simulink model "Pendule_Observateur_Controleur_Discret"  (Simulink 8.4)
settings: Solver=ode3  StartTime=0.0  StopTime=10.0  RelTol=1e-3
values from neighbouring files (symbols this model uses):
  A = zeros (4,4)    [Modele_Pendule.m]
  Aod = Ad-Kod*Cd    [Design_Matlab_File_Pendule_IMC_.m]
  B = zeros (4,1)    [Modele_Pendule.m]
  Bod = [Bd Kod]    [Design_Matlab_File_Pendule_IMC_.m]
  C = [1 0 0 0 ... (first row only)    [Modele_Pendule.m]
  Cod = eye(4,4)    [Design_Matlab_File_Pendule_IMC_.m]
  D = [ 0 0 ]'    [Modele_Pendule.m]
  Dod = zeros(4,3)    [Design_Matlab_File_Pendule_IMC_.m]
  Kcd = place(Ad,Bd,Pcd)    [Design_Matlab_File_Pendule_IMC_.m]
  T_ech = 0.005    [Design_Matlab_File_Pendule_IMC_.m]
  X0 = [0.3 0 0 0]'    [Design_Matlab_File_Pendule_IMC_.m]
libraries: simulink_extras x1
settings Model: Creator=reama  LastModifiedBy=ArbenCela
settings OptimizationCC: InitFltsAndDblsToZero=on
settings DebuggingCC: SaveWithParameterizedLinksMsg=none  SignalResolutionControl=TryResolveAllWithWarning  MultiTaskDSMMsg=warning  MultiTaskCondExecSysMsg=none
settings RTWCC: IncludeERTFirstTime=on
settings GRTTargetCC: TargetFcnLib=ansi_tfl_tmw.mat

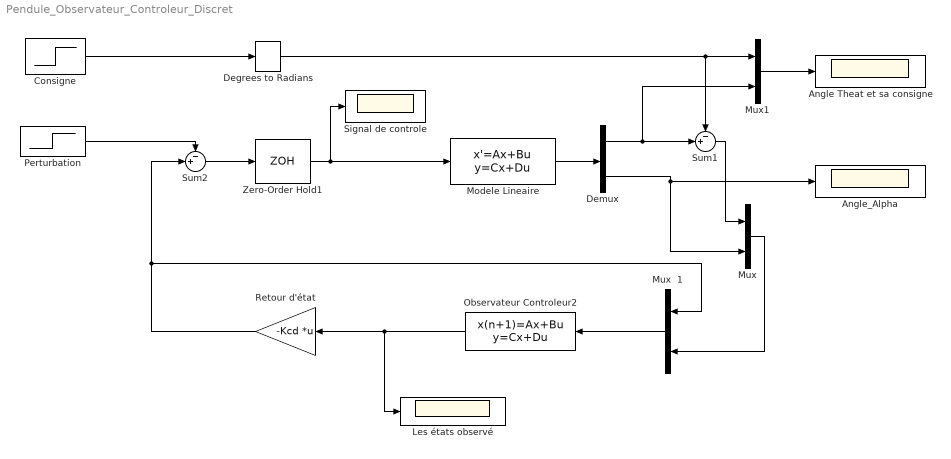
== system Pendule_Observateur_Controleur_Discret ==
  Angle Theat et sa consigne : Scope
      settings: SaveName=ScopeData5
  Angle_Alpha : Scope
  Consigne : Step  Time=6  After=50  SampleTime=0
  Degrees to Radians : simulink_extras/Transformations/Degrees to Radians
  Demux : Demux  Outputs=2
  Les états observé : Scope
      settings: SaveName=ScopeData3
  Modele Lineaire : StateSpace  A=A  B=B  C=C  D=D  X0=X0
  Mux : Mux  Inputs=2
  Mux  1 : Mux  Inputs=2
  Mux1 : Mux  Inputs=2
  Observateur Controleur2 : DiscreteStateSpace  A=Aod  B=Bod  C=Cod  D=Dod  SampleTime=T_ech
  Perturbation : Step  Time=6  SampleTime=0
  "Retour d'état " : Gain  Gain=-Kcd  Multiplication=Matrix(K*u)  SaturateOnIntegerOverflow=on  OutDataTypeStr=Inherit: Same as input  ParamDataTypeStr=Inherit: Same as input
  Signal de controle : Scope
  Sum1 : Sum  Inputs=-+|  SaturateOnIntegerOverflow=on  InputSameDT=on  OutDataTypeStr=Inherit: Same as first input
  Sum2 : Sum  Inputs=-+|  SaturateOnIntegerOverflow=on  InputSameDT=on  OutDataTypeStr=Inherit: Same as first input
  Zero-Order Hold1 : ZeroOrderHold  SampleTime=T_ech
  wires:
  Modele Lineaire/1 -> Demux/1
  Demux/2 -> Mux/2, Angle_Alpha/1
  Degrees to Radians/1 -> Mux1/1, Sum1/1
  Consigne/1 -> Degrees to Radians/1
  Demux/1 -> Mux1/2, Sum1/2
  Sum1/1 -> Mux/1
  Observateur Controleur2/1 -> Les états observé/1, "Retour d'état "/1
  Mux  1/1 -> Observateur Controleur2/1
  "Retour d'état "/1 -> Sum2/2, Mux  1/1
  Zero-Order Hold1/1 -> Modele Lineaire/1, Signal de controle/1
  Mux1/1 -> Angle Theat et sa consigne/1
  Mux/1 -> Mux  1/2
  Sum2/1 -> Zero-Order Hold1/1
  Perturbation/1 -> Sum2/1
